simulink model "traitement_LPC"  (Simulink 7.4)
settings: Solver=FixedStepDiscrete  SolverMode=SingleTasking  StartTime=0.0  StopTime=inf  RelTol=1e-3
PreLoadFcn:
  | load mtlb;
undefined symbols (not defined in the file or in its folder): dfilt
libraries: dspstat3 x1, dspbuff3 x1, dspsigops x1, dspsolvers x1, dsparch4 x1, dspsrcs4 x1
settings Model: RequirementInfo=9  Creator=dshpak  LastModifiedBy=Nayve  CovMetricSettings=d  ExtModeTrigMode=oneshot  ExtModeArmWhenConnect=off  ExtModeAutoUpdateStatusClock=off
settings DataIOCC: LimitDataPoints=off  SaveFormat=Structure  SaveOutput=off  SaveTime=off  SignalLoggingName=sigsOut
settings OptimizationCC: BlockReduction=off  BooleanDataType=off
settings DebuggingCC: SaveWithParameterizedLinksMsg=none  SignalResolutionControl=TryResolveAllWithWarning  SolverPrmCheckMsg=none  MultiTaskDSMMsg=warning  MultiTaskCondExecSysMsg=none  IntegerOverflowMsg=none  StrictBusMsg=None
settings HardwareCC: TargetUnknown=on
settings RTWCC: IncludeERTFirstTime=on

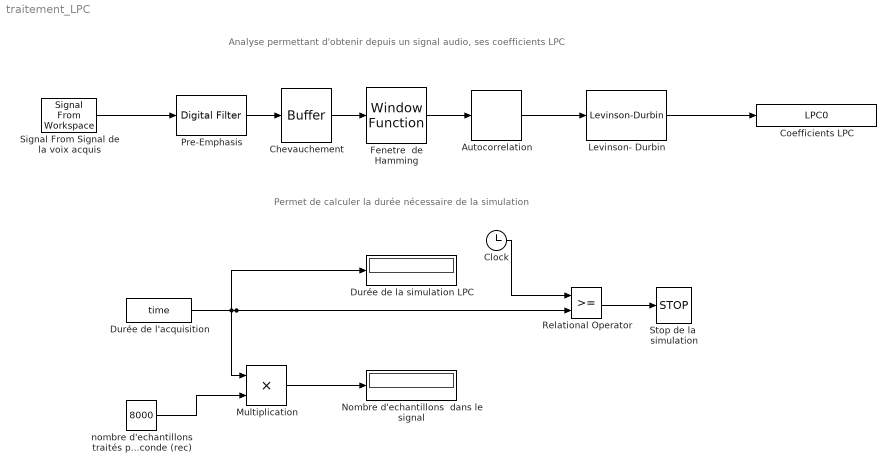
== system traitement_LPC ==
  note: Analyse permettant d'obtenir depuis un signal audio, ses coefficients LPC
  note: Permet de calculer la durée nécessaire de la simulation
  Autocorrelation : dspstat3/Autocorrelation  DialogController=dspDDGCreate  DialogControllerArgs=DataTag0  AllPositiveLags=off  maxlag=12  bias=Biased  domain=Time  outputDataTypeStr=Inherit: Same as accumulator  outputLastDataTypeStr=Inherit: Same as accumulator  outputMin=[]  outputMax=[]  roundingMode=Floor  overflowMode=off
  Chevauchement : dspbuff3/Buffer  N=160  V=80  ic=0
  Clock : Clock
      settings: Decimation=10
  Coefficients LPC : ToWorkspace  VariableName=LPC0  SampleTime=-1  SaveFormat=Array
  Durée de l'acquisition : FromWorkspace  VariableName=time  SampleTime=0
  Durée de la simulation LPC : Display
  Fenetre  de Hamming : dspsigops/Window Function  DialogController=dspDDGCreate  DialogControllerArgs=DataTag1  winmode=Apply window to input  wintype=Hamming  sampmode=Continuous  samptime=1  N=64  Rs=50  beta=10  winsamp=Symmetric  UserWindow=hamming  OptParams=off  UserParams={1.0}  dataType=double  isSigned=on  wordLen=16  udDataType=sfix(16)  fracBitsMode=Best precision  numFracBits=15  roundingMode=Floor  overflowMode=off  numSidelobes=4  sidelobeLevel=-30
  Levinson- Durbin : dspsolvers/Levinson-Durbin  DialogController=dspDDGCreate  DialogControllerArgs=DataTag2  coeffOutFcn=OBSOLETE  coeffOutFcnActive=A  outP=off  zeroInpHandling=on  firstCoeffMode=Binary point scaling  firstCoeffWordLength=16  firstCoeffFracLength=15  firstCoeffDataTypeStr=fixdt(1,16,15)  firstCoeffLastDataTypeStr=fixdt(1,16,15)  firstCoeffMin=[]  firstCoeffMax=[]  secondCoeffMode=Binary point scaling  secondCoeffWordLength=16  secondCoeffFracLength=15  secondCoeffDataTypeStr=fixdt(1,16,15)  secondCoeffLastDataTypeStr=fixdt(1,16,15)  secondCoeffMin=[]  secondCoeffMax=[]  outputMin=[]  outputMax=[]  roundingMode=Floor  overflowMode=off
      settings: allowOverrides=off
  Multiplication : Product  Inputs=**  OutDataTypeMode=single  OutDataType=sfix(16)  OutScaling=2^-10  OutDataTypeStr=single
  "Nombre d'echantillons  dans le signal " : Display
  Pre-Emphasis : dsparch4/Digital Filter  DialogController=dspdialog.DigitalFilter  DialogControllerArgs=DataTag3  TypePopup=FIR (all zeros)  IIRFiltStruct=Direct form II transposed  AllPoleFiltStruct=Direct form  FIRFiltStruct=Direct form  CoeffSource=Specify via dialog  NumCoeffs=[1 -.95]  DenCoeffs=[1 0.1]  BiQuadCoeffs=[1 0.3 0.4 1 0.1 0.2]  LatticeCoeffs=[0.2 0.4]  denIgnore=on  FiltPerSampPopup=One filter per frame  IC=0  ICnum=0  ICden=0  roundingMode=Floor  overflowMode=off  ScaleValues=1  scaleValueFracLength=14  stageInFracLength=15  stageOutFracLength=15  FilterSource=Specify via dialog  dfiltObjectName=dfilt.dffir([1 2 1])
  Relational Operator : RelationalOperator
  Signal From Signal de la voix acquis : dspsrcs4/Signal From Workspace  SystemSampleTime=-1  X=voix  Ts=1/8000  nsamps=160  OutputAfterFinalValue=Setting to zero  ignoreOrWarnInputAndFrameLengths=off
  Stop de la  simulation : Stop
  nombre d'echantillons traités par seconde (rec) : Constant  Value=8000  OutDataTypeMode=double  OutDataType=sfix(16)  OutScaling=2^0  OutDataTypeStr=double
  wires:
  Signal From Signal de la voix acquis/1 -> Pre-Emphasis/1
  Pre-Emphasis/1 -> Chevauchement/1
  Levinson- Durbin/1 -> Coefficients LPC/1
  Autocorrelation/1 -> Levinson- Durbin/1
  Fenetre  de Hamming/1 -> Autocorrelation/1
  Chevauchement/1 -> Fenetre  de Hamming/1
  Clock/1 -> Relational Operator/1
  Relational Operator/1 -> Stop de la  simulation/1
  nombre d'echantillons traités par seconde (rec)/1 -> Multiplication/2
  Multiplication/1 -> "Nombre d'echantillons  dans le signal "/1
  Durée de l'acquisition/1 -> Relational Operator/2, Multiplication/1, Durée de la simulation LPC/1
